simulink model "GH2_prop_valve_tuner"  (R2024b)
settings: Solver=ode15s  StartTime=0.0  StopTime=inf  RelTol=1e-3
settings Model: Creator=MW  LastModifiedBy=MW

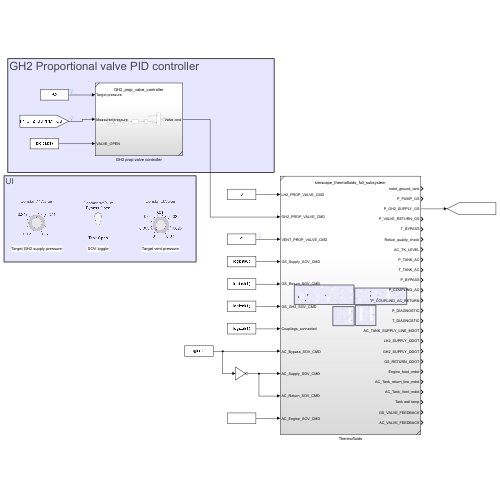
[thumbnail: Simulink's stored preview of the top-level diagram]
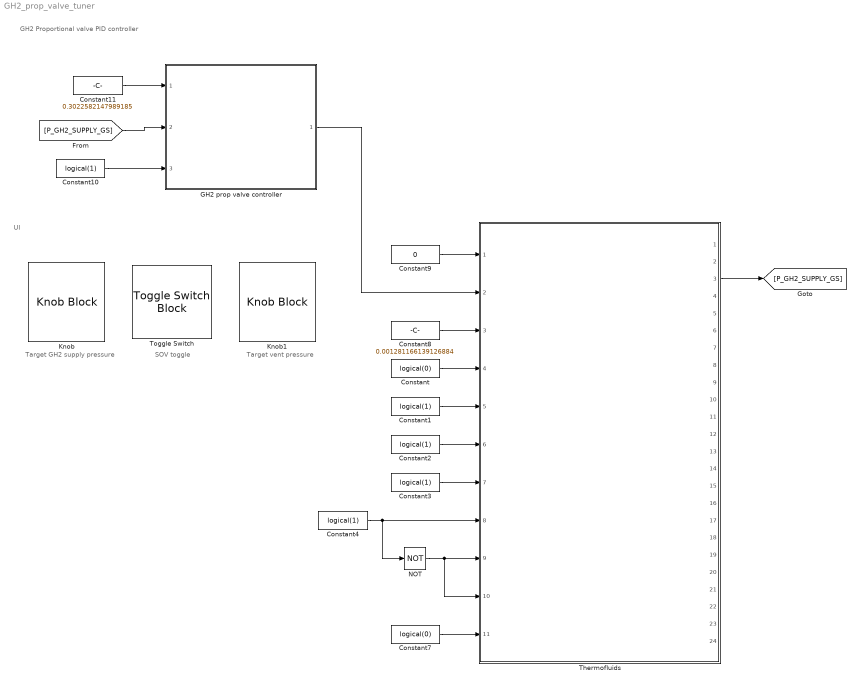
== system GH2_prop_valve_tuner ==
  note: Target GH2 supply pressure
  note: UI
  note: GH2 Proportional valve PID controller
  note: Target vent pressure
  note: SOV toggle
  Constant : Constant  Value=logical(0)
  Constant{1..4,10} (5 alike) : Constant  Value=logical(1)
  Constant11 : Constant  Value=0.3022582147989185
  Constant7 : Constant  Value=logical(0)
  Constant8 : Constant  Value=0.001281166139126884
  Constant9 : Constant  Value=0
  GH2 prop valve controller : Subsystem  ReferencedSubsystem=GH2_prop_valve_controller
  Knob : KnobBlock  ScaleMin=0.12  ScaleMax=0.5
  Knob1 : KnobBlock  ScaleMax=0.03
  NOT : Logic  Operator=NOT  IconShape=distinctive  AllPortsSameDT=off  OutDataTypeStr=boolean
  Thermofluids : Subsystem  ReferencedSubsystem=simscape_thermofluids_full_subsystem
  Toggle Switch : ToggleSwitchBlock
      settings: Values={{'Tank Open', 'Bypass Open'}, [0 1]}
  wires:
  Constant/1 -> Thermofluids/4
  Constant1/1 -> Thermofluids/5
  Constant2/1 -> Thermofluids/6
  Constant3/1 -> Thermofluids/7
  Constant4/1 -> NOT/1, Thermofluids/8
  NOT/1 -> Thermofluids/9, Thermofluids/10
  Constant7/1 -> Thermofluids/11
  Constant8/1 -> Thermofluids/3
  Constant11/1 -> GH2 prop valve controller/1
  Constant10/1 -> GH2 prop valve controller/3
  [P_GH2_SUPPLY_GS] -> GH2 prop valve controller/2
  Thermofluids/3 -> [P_GH2_SUPPLY_GS]
  Constant9/1 -> Thermofluids/1
  GH2 prop valve controller/1 -> Thermofluids/2
